simulink model "drone_ilc"  (R2019a)
settings: Solver=VariableStepAuto  StartTime=0.0  StopTime=inf  RelTol=1e-3
libraries: robotlib x2, simulink_need_slupdate x1, aerolibanimutils x1
settings Model: Creator=flying  LastModifiedBy=flying

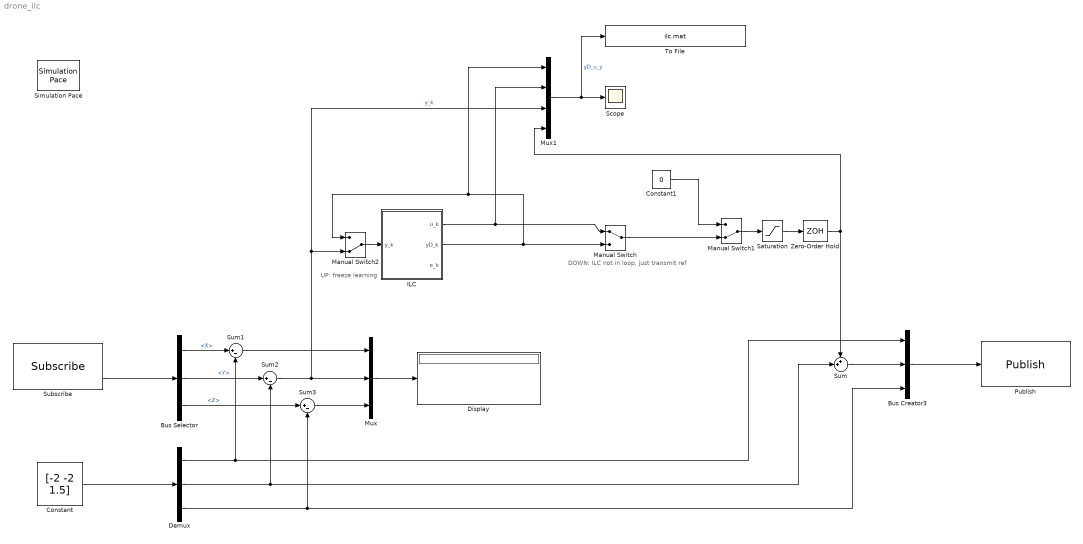
== system drone_ilc ==
  note: UP: freeze learning
  note: DOWN: ILC not in loop, just transmit ref
  Bus Creator3 : BusCreator  Inputs=3  OutDataTypeStr=Bus: SL_Bus_drone_ilc_geometry_msgs_Vector3  NonVirtualBus=on
      settings: InheritFromInputs=off
  Bus Selector : BusSelector  OutputSignals=Transform.Translation.X,Transform.Translation.Y,Transform.Translation.Z
  Constant : Constant  Value=[-2 -2 1.5]
  Constant1 : Constant  Value=0
  Demux : Demux  Outputs=3
  Display : Display
  ILC : Subsystem  Description=Iterative Learning Control  TreatAsAtomicUnit=on  SystemSampleTime=dt  mask(Iterative Learning Control){Yseq=[sin((0:40)*2*pi/160).^3 1-0.5*sin((0:40)*2*pi/160).^3 0.5+0.5*sin((0:40)*2*pi/160).^3 1-sin((0:40)*2*pi/160).^3], dt=0.2, gamma=0.16, offset=20}
      mask prompts: Yseq "Desired output sequence"; dt "Time step"; gamma "Learning rate"; offset "Learning offset"
      mask help:
      | Adapts the applied input u such that the system output y tracks the desired output sequence yDes.
      |
      | Update equation is u(k+N-p)=u(k)+g*e(k) where N is the sequence length, p is the learning offset, g is the learning rate and e is the error, e(k)=yDes(k)-y(k).
  Manual Switch : ManualSwitch
  Manual Switch1 : ManualSwitch  CurrentSetting=0
  Manual Switch2 : ManualSwitch  CurrentSetting=0
  Mux : Mux  Inputs=3
  Mux1 : Mux
  Publish : robotlib/Publish  topicSource=Select from ROS network  topic=/input_pos  messageType=geometry_msgs/Vector3  messageQueueLength=1
      settings: SourceProductBaseCode=RO
  Saturation : Saturate  UpperLimit=2  LowerLimit=-2
  Scope : Scope
  Simulation Pace : aerolibanimutils/Simulation Pace  SimulationPace=1  SleepMode=Auto  OutputPaceError=off  SampleTime=1/30
  Subscribe : robotlib/Subscribe  topicSource=Select from ROS network  topic=/vicon/Debbie/Debbie  messageType=geometry_msgs/TransformStamped  sampleTime=0.2  messageQueueLength=1
      settings: SourceProductBaseCode=RO
  Sum : Sum  Inputs=++|
  Sum1 : Sum  Inputs=|+-
  Sum2 : Sum  Inputs=|+-
  Sum3 : Sum  Inputs=|+-
  To File : ToFile  Filename=ilc.mat  MatrixName=ilc_result  SaveFormat=Timeseries
  Zero-Order Hold : ZeroOrderHold  SampleTime=0.1
  wires:
  Bus Creator3/1 -> Publish/1
  Constant/1 -> Demux/1
  Demux/3 -> Sum3/2, Bus Creator3/3
  Subscribe/2 -> Bus Selector/1
  ILC/1(u_k) -> Mux1/2, Manual Switch/1
  Saturation/1 -> Zero-Order Hold/1
  Demux/2 -> Sum2/2, Sum/2
  Sum/1 -> Bus Creator3/2
  Manual Switch1/1 -> Saturation/1
  Manual Switch/1 -> Manual Switch1/2
  Constant1/1 -> Manual Switch1/1
  Mux/1 -> Display/1
  Manual Switch2/1 -> ILC/1(y_k)
  ILC/2(yD_k) -> Mux1/1, Manual Switch2/1, Manual Switch/2
  Zero-Order Hold/1 -> Mux1/4, Sum/1
  Bus Selector/1 -> Sum1/1  "<X>"
  Sum1/1 -> Mux/1
  Demux/1 -> Sum1/2, Bus Creator3/1
  Bus Selector/2 -> Sum2/1  "<Y>"
  Sum2/1 -> Mux1/3, Manual Switch2/2, Mux/2  "y_k"
  Sum3/1 -> Mux/3
  Bus Selector/3 -> Sum3/1  "<Z>"
  Mux1/1 -> To File/1, Scope/1  "yD_u_y"

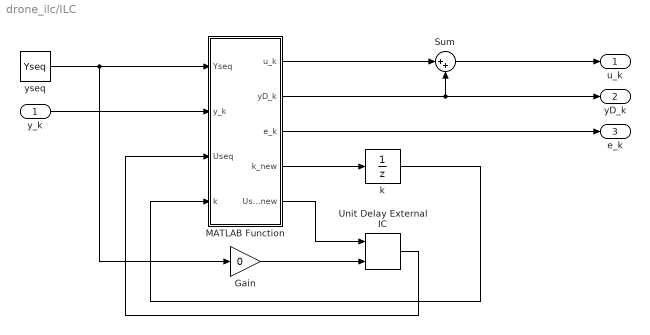
== system drone_ilc/ILC ==
  y_k : Inport
  Gain : Gain  Gain=0
  MATLAB Function : MATLAB Function  TreatAsAtomicUnit=on
  Sum : Sum  Inputs=|++
  Unit Delay External IC : simulink_need_slupdate/Unit Delay External IC  tsamp=-1
      settings: SourceProductName=Simulink  SourceProductBaseCode=SL
  k : UnitDelay  InitialCondition=1  SampleTime=-1  HasFrameUpgradeWarning=on
  yseq : Constant  Value=Yseq
  u_k : Outport
  yD_k : Outport  Port=2
  e_k : Outport  Port=3
  wires:
  MATLAB Function/4(k_new) -> k/1
  MATLAB Function/5(Useq_new) -> Unit Delay External IC/1
  Unit Delay External IC/1 -> MATLAB Function/3(Useq)
  y_k/1 -> MATLAB Function/2(y_k)
  yseq/1 -> MATLAB Function/1(Yseq), Gain/1
  k/1 -> MATLAB Function/4(k)
  MATLAB Function/2(yD_k) -> yD_k/1, Sum/2
  Sum/1 -> u_k/1
  MATLAB Function/1(u_k) -> Sum/1
  Gain/1 -> Unit Delay External IC/2
  MATLAB Function/3(e_k) -> e_k/1

== matlab function drone_ilc/ILC/MATLAB Function ==
  data: u_k output; Yseq input; yD_k output; e_k output; y_k input; Useq input; k input; k_new output; Useq_new output; gamma parameter; offset parameter
function [u_k,yD_k,e_k,k_new,Useq_new] = fcn(Yseq,y_k,Useq,k,gamma,offset)
%#codegen

% number of elements in sequence
Nseq = numel(Yseq);

% counter
k_new = k+1;
% reset if we've been round the sequence
if k_new>Nseq,
    k_new=1;
end

% extract current demand signal
yD_k = Yseq(k);

% and the current control
u_k = Useq(k);

% form the error
e_k = yD_k - y_k;

% copy the control sequence over
Useq_new = Useq;

% which entry to update
k_learn = k-offset;
while k_learn<1
    k_learn=k_learn+Nseq;
end

% do the learning update
Useq_new(k_learn) = Useq_new(k_learn) + gamma*e_k;
